simulink model "system_sim"  (R2023b)
settings: Solver=VariableStepAuto  StartTime=0.0  StopTime=10.0  RelTol=1e-3
undefined symbols (not defined in the file): ct_A, ct_B, ct_C, ct_D, F, G, H, J, ts, xp_init
settings Model: Creator=mike5  LastModifiedBy=mike5

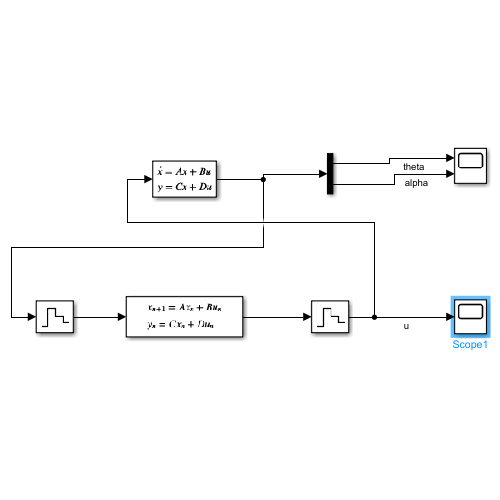
[thumbnail: Simulink's stored preview of the top-level diagram]
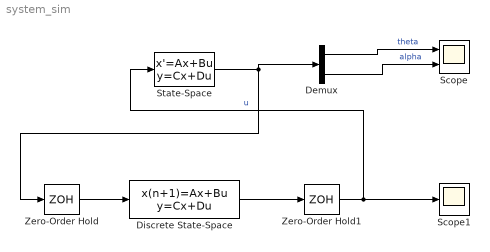
== system system_sim ==
  Demux : Demux  Outputs=2
  Discrete State-Space : DiscreteStateSpace  A=F  B=G  C=H  D=J  SampleTime=-1
  Scope : Scope  NumInputPorts=2
  Scope1 : Scope
  State-Space : StateSpace  A=ct_A  B=ct_B  C=ct_C  D=ct_D  InitialCondition=xp_init
  Zero-Order Hold : ZeroOrderHold  SampleTime=ts
  Zero-Order Hold1 : ZeroOrderHold  SampleTime=-1
  wires:
  Zero-Order Hold/1 -> Discrete State-Space/1
  Discrete State-Space/1 -> Zero-Order Hold1/1
  State-Space/1 -> Demux/1, Zero-Order Hold/1
  Zero-Order Hold1/1 -> State-Space/1, Scope1/1  "u"
  Demux/1 -> Scope/1  "theta"
  Demux/2 -> Scope/2  "alpha"
